simulink model "Substructuring"  (R2021a)
settings: Solver=ode8  StartTime=0.0  StopTime=31.2  FixedStep=dtfast  RelTol=1e-3
PreLoadFcn:
  | initializeSimulation;
InitFcn:
  | clear('all');
  | initializeSimulation;
undefined symbols (not defined in the file): adaptive, Ap, asiv, Bp, Cp, DiscIntNeverNeededParam, Dp, dtsim, f, ke, kgap, khard, learningrate, n1siv, n2siv, Ngap, nsiv, stiffdeg, strdegHmos, V1, w_80, x02, xgap, xy
libraries: raspberrypiNetworklib x2, instrumentlib x2, sldrtlib x1
settings Model: Creator=diego.mera  LastModifiedBy=diego.mera
settings SolverCC: PositivePriorityOrder=on
settings OptimizationCC: EnhancedBackFolding=on  PassReuseOutputArgsAs=Individual arguments  ZeroExternalMemoryAtStartup=off  ZeroInternalMemoryAtStartup=off  MaxStackSize=64  OptimizeBlockOrder=speed  DifferentSizesBufferReuse=on  OptimizationCustomize=off  EfficientTunableParamExpr=on
settings DebuggingCC: ParameterTunabilityLossMsg=error
settings HardwareCC: ProdBitPerPointer=32  ProdBitPerSizeT=32  ProdBitPerPtrDiffT=32  ProdLargestAtomicInteger=Long  ProdLargestAtomicFloat=Double  ProdWordSize=32  ProdLongLongMode=on  ProdHWDeviceType=ARM Compatible->ARM Cortex
settings RTWCC: SystemTargetFile=ert.tlc  HardwareBoard=Raspberry Pi  TLCOptions="-aInlineSetEventsForThisBaseRateFcn=TLC_FALSE -aSuppressMultiTaskScheduler=TLC_FALSE  -aRateBasedStepFcn=0"  TemplateMakefile=ert_default_tmf  Toolchain=GNU GCC Embedded Linux  BuildConfiguration=Faster Runs
settings CodeAppCC: ForceParamTrailComments=on  IgnoreCustomStorageClasses=off  OperatorAnnotations=on  SimulinkDataObjDesc=on  SFDataObjDesc=on  InsertBlockDesc=on
settings ERTTargetCC: SupportContinuousTime=on  SupportVariableSizeSignals=on  ExtModeTransport=2  ExtModeStaticAlloc=on  ExtModeMexFile=ext_xcp  ExtModeIntrfLevel=Level2 - Open

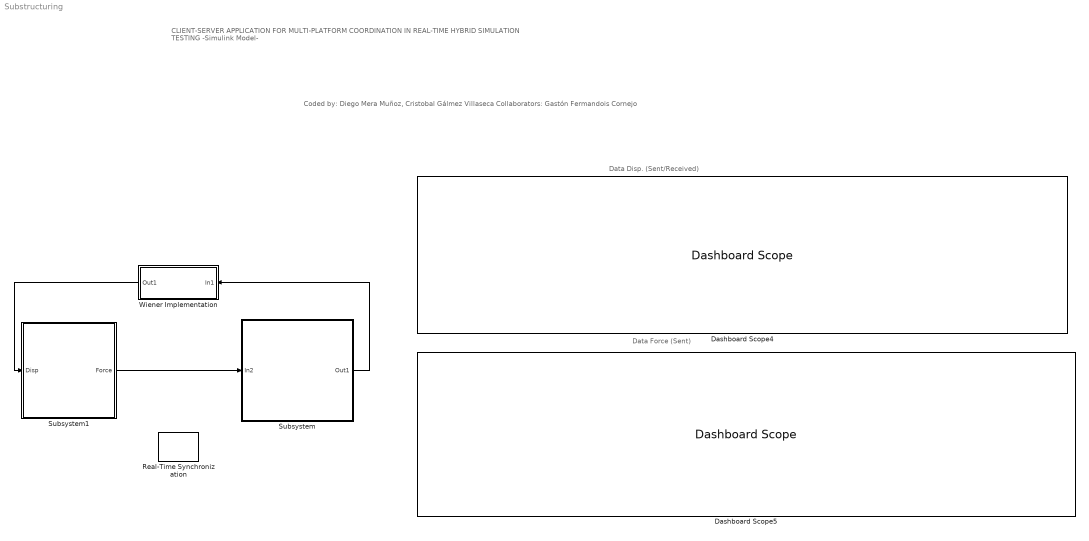
== system Substructuring ==
  note: Data Disp. (Sent/Received)
  note: Data Force (Sent)
  note: CLIENT-SERVER APPLICATION FOR MULTI-PLATFORM COORDINATION IN REAL-TIME HYBRID SIMULATION TESTING
      | -Simulink Model-
  note: Coded by: Diego Mera Muñoz, Cristobal Gálmez Villaseca
      | Collaborators: Gastón Fermandois Cornejo
  Dashboard Scope4 : DashboardScope  Ymin=-5  Ymax=5
  Dashboard Scope5 : DashboardScope  Ymin=-1.5e-5  Ymax=1e-5
  Real-Time Synchronization : sldrtlib/Real-Time Synchronization  SampleTime=dtsim  MaxMissedTicks=1000000  ShowMissedTicks=off  YieldWhenWaiting=off
  Subsystem : Subsystem
      mask Display: disp('NUMERICAL\nSUBSTRUCTURE')
  Subsystem1 : Subsystem
      mask Display: disp('EXPERIMENTAL\nSUBSTRUCTURE')
  Wiener Implementation : Subsystem
      mask Display: disp('DDMRT FILTER')
  wires:
  Subsystem1/1(Force) -> Subsystem/1(In2)
  Subsystem/1(Out1) -> Wiener Implementation/1(In1)
  Wiener Implementation/1(Out1) -> Subsystem1/1(Disp)

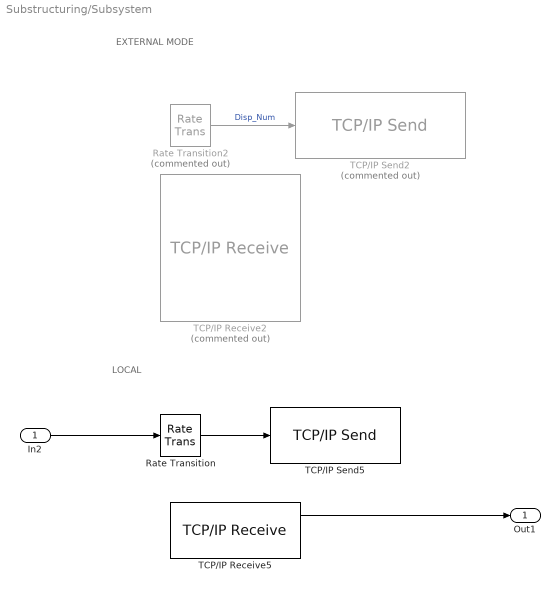
== system Substructuring/Subsystem ==
  note: EXTERNAL MODE
  note: LOCAL
  In2 : Inport
  Rate Transition : RateTransition  OutPortSampleTime=dtsim
  Rate Transition2 : RateTransition  Commented=on  OutPortSampleTime=dtsim
  TCP/IP Receive2 : raspberrypiNetworklib/TCP//IP Receive  Priority=2  Commented=on  Mode_=Client  LocalServerPort_=8090  RemoteAddr_=192.168.0.18  RemoteServerPort_=8090  DataType_=double  DataSize_=1  SampleTime_=dtsim  SimulateUsing=Code generation  ClientPortBindingSelection_=off  ClientPortToBind_=35000  BlockingMode_=on  BlockTimeout_=0.01  BlockPlatform=RASPBERRYPI
      settings: SourceProductBaseCode=RASPPI
  TCP/IP Receive5 : instrumentlib/TCP//IP Receive  Priority=1  Host=127.0.0.1  Port=8090  DataSize=1  EnableBlockingMode=off  Timeout=10  SampleTime=dtsim  DataType=double  ByteOrder=BigEndian  ASCIIFormatting=%f,  Terminator=LF
  TCP/IP Send2 : raspberrypiNetworklib/TCP//IP Send  Priority=1  Commented=on  Mode_=Client  LocalServerPort_=8090  RemoteAddr_=192.168.0.18  RemoteServerPort_=8090  SimulateUsing=Code generation  ClientPortBindingSelection_=off  ClientPortToBind_=35000  BlockingMode_=on  BlockTimeout_=0.02  BlockPlatform=RASPBERRYPI
      settings: SourceProductBaseCode=RASPPI
  TCP/IP Send5 : instrumentlib/TCP//IP Send  Priority=2  Host=127.0.0.1  Port=8090  EnableBlockingMode=off  Timeout=0.02  ByteOrder=BigEndian  TransferDelay=on
  Out1 : Outport
  wires:
  Rate Transition/1 -> TCP/IP Send5/1
  Rate Transition2/1 -> TCP/IP Send2/1  "Disp_Num"
  In2/1 -> Rate Transition/1
  TCP/IP Receive5/1 -> Out1/1

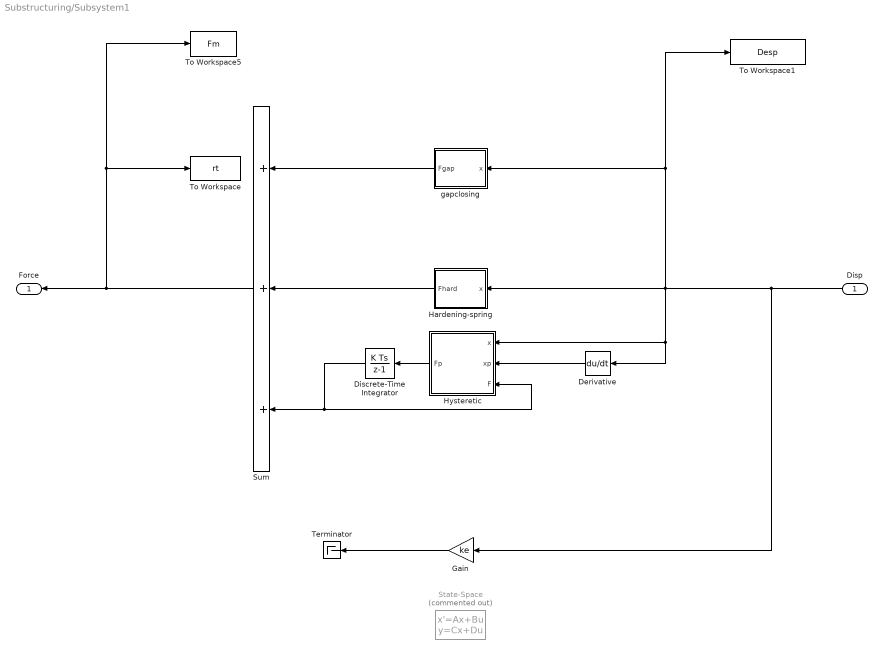
== system Substructuring/Subsystem1 ==
  Disp : Inport
  Derivative : Derivative
  Discrete-Time Integrator : DiscreteIntegrator  SampleTime=-1  ICPrevOutput=DiscIntNeverNeededParam  ICPrevScaledInput=DiscIntNeverNeededParam
  Gain : Gain  Gain=ke
  Hardening-spring : Subsystem
  Hysteretic : Subsystem
  State-Space : StateSpace  Commented=on  A=Ap  B=Bp  C=Cp  D=Dp  InitialCondition=0
  Sum : Sum  Inputs=+++
  Terminator : Terminator
  To Workspace : ToWorkspace  VariableName=rt  SaveFormat=Timeseries  SampleTime=-1
  To Workspace1 : ToWorkspace  VariableName=Desp  SaveFormat=Timeseries  SampleTime=-1
  To Workspace5 : ToWorkspace  VariableName=Fm  SaveFormat=Timeseries  SampleTime=-1
  gapclosing : Subsystem
  Force : Outport  VectorParamsAs1DForOutWhenUnconnected=off
  wires:
  gapclosing/1(Fgap) -> Sum/1
  Discrete-Time Integrator/1 -> Hysteretic/3(F), Sum/3
  Hardening-spring/1(Fhard) -> Sum/2
  Hysteretic/1(Fp) -> Discrete-Time Integrator/1
  Derivative/1 -> Hysteretic/2(xp)
  Disp/1 -> Gain/1, To Workspace1/1, gapclosing/1(x), Hysteretic/1(x), Derivative/1, Hardening-spring/1(x)
  Sum/1 -> To Workspace5/1, To Workspace/1, Force/1
  Gain/1 -> Terminator/1

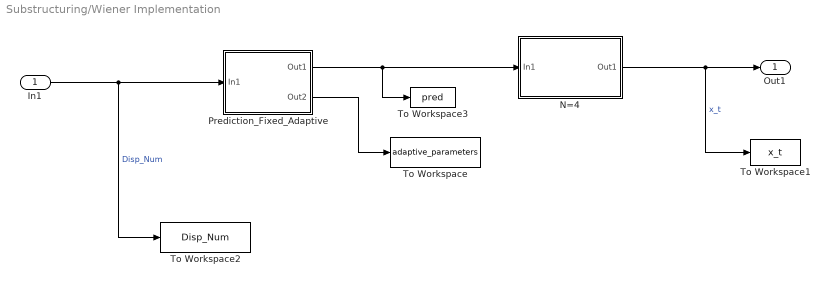
== system Substructuring/Wiener Implementation ==
  In1 : Inport
  N=4 : Subsystem
      mask Display: disp('MONOMIAL\nINTERPOLATION')
  Prediction_Fixed_Adaptive : Subsystem
      mask Display: disp('PREDICTION\n(Adaptive w)')
  To Workspace : ToWorkspace  VariableName=adaptive_parameters  SaveFormat=Timeseries  SampleTime=-1
  To Workspace1 : ToWorkspace  VariableName=x_t  SaveFormat=Timeseries  SampleTime=-1
  To Workspace2 : ToWorkspace  VariableName=Disp_Num  SaveFormat=Timeseries  SampleTime=-1
  To Workspace3 : ToWorkspace  VariableName=pred  SaveFormat=Timeseries  SampleTime=-1
  Out1 : Outport
  wires:
  In1/1 -> Prediction_Fixed_Adaptive/1(In1), To Workspace2/1  "Disp_Num"
  Prediction_Fixed_Adaptive/2(Out2) -> To Workspace/1
  N=4/1(Out1) -> To Workspace1/1, Out1/1  "x_t"
  Prediction_Fixed_Adaptive/1(Out1) -> To Workspace3/1, N=4/1(In1)

== system Substructuring/Subsystem1/Hardening-spring ==
  x : Inport
  Constant1 : Constant  Value=khard
  MATLAB Function : MATLAB Function  TreatAsAtomicUnit=on
  To Workspace : ToWorkspace  VariableName=Fhard  SaveFormat=Timeseries  SampleTime=-1
  Unit Delay : UnitDelay  SampleTime=-1  HasFrameUpgradeWarning=on
  Fhard : Outport  VectorParamsAs1DForOutWhenUnconnected=off
  wires:
  x/1 -> Unit Delay/1
  Constant1/1 -> MATLAB Function/2(khard)
  MATLAB Function/1(Fhard) -> Fhard/1, To Workspace/1
  Unit Delay/1 -> MATLAB Function/1(x)

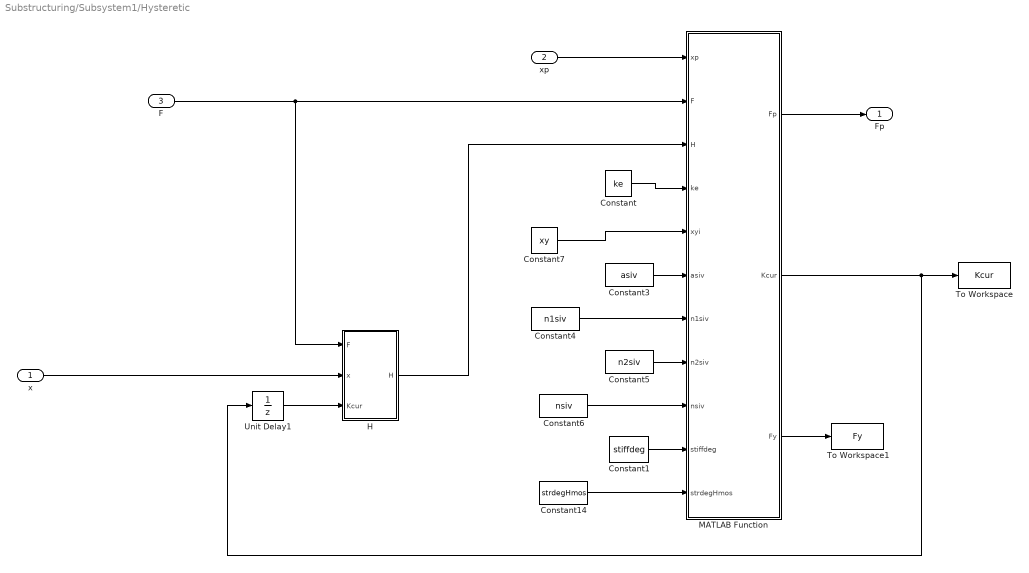
== system Substructuring/Subsystem1/Hysteretic ==
  x : Inport
  xp : Inport  Port=2
  F : Inport  Port=3
  Constant : Constant  Value=ke
  Constant1 : Constant  Value=stiffdeg
  Constant14 : Constant  Value=strdegHmos
  Constant3 : Constant  Value=asiv
  Constant4 : Constant  Value=n1siv
  Constant5 : Constant  Value=n2siv
  Constant6 : Constant  Value=nsiv
  Constant7 : Constant  Value=xy
  H : Subsystem
  MATLAB Function : MATLAB Function  TreatAsAtomicUnit=on
  To Workspace : ToWorkspace  VariableName=Kcur  SaveFormat=Timeseries  SampleTime=-1
  To Workspace1 : ToWorkspace  VariableName=Fy  SaveFormat=Timeseries  SampleTime=-1
  Unit Delay1 : UnitDelay  InitialCondition=ke  SampleTime=-1  HasFrameUpgradeWarning=on
  Fp : Outport  VectorParamsAs1DForOutWhenUnconnected=off
  wires:
  MATLAB Function/1(Fp) -> Fp/1
  MATLAB Function/2(Kcur) -> To Workspace/1, Unit Delay1/1
  x/1 -> H/2(x)
  xp/1 -> MATLAB Function/1(xp)
  Constant/1 -> MATLAB Function/4(ke)
  Constant7/1 -> MATLAB Function/5(xyi)
  Constant1/1 -> MATLAB Function/10(stiffdeg)
  Constant3/1 -> MATLAB Function/6(asiv)
  Constant4/1 -> MATLAB Function/7(n1siv)
  Constant5/1 -> MATLAB Function/8(n2siv)
  Constant6/1 -> MATLAB Function/9(nsiv)
  H/1(H) -> MATLAB Function/3(H)
  Unit Delay1/1 -> H/3("Kcur ")
  F/1 -> MATLAB Function/2(F), H/1(F)
  MATLAB Function/3(Fy) -> To Workspace1/1
  Constant14/1 -> MATLAB Function/11(strdegHmos)

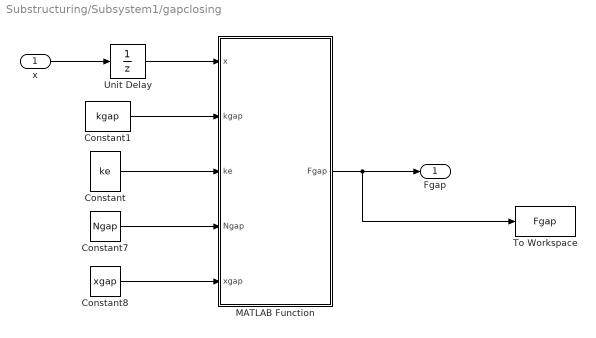
== system Substructuring/Subsystem1/gapclosing ==
  x : Inport
  Constant : Constant  Value=ke
  Constant1 : Constant  Value=kgap
  Constant7 : Constant  Value=Ngap
  Constant8 : Constant  Value=xgap
  MATLAB Function : MATLAB Function  TreatAsAtomicUnit=on
  To Workspace : ToWorkspace  VariableName=Fgap  SaveFormat=Timeseries  SampleTime=-1
  Unit Delay : UnitDelay  SampleTime=-1  HasFrameUpgradeWarning=on
  Fgap : Outport  VectorParamsAs1DForOutWhenUnconnected=off
  wires:
  Constant7/1 -> MATLAB Function/4(Ngap)
  MATLAB Function/1(Fgap) -> To Workspace/1, Fgap/1
  Constant1/1 -> MATLAB Function/2(kgap)
  Constant8/1 -> MATLAB Function/5(xgap)
  Constant/1 -> MATLAB Function/3(ke)
  x/1 -> Unit Delay/1
  Unit Delay/1 -> MATLAB Function/1(x)

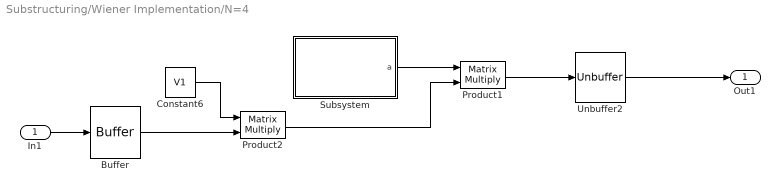
== system Substructuring/Wiener Implementation/N=4 ==
  In1 : Inport
  Buffer : Buffer  N=4  V=3  OutputFrames=off
  Constant6 : Constant  Value=V1
  Product1 : Product  Multiplication=Matrix(*)
  Product2 : Product  Multiplication=Matrix(*)
  Subsystem : Subsystem
  Unbuffer2 : Unbuffer
  Out1 : Outport
  wires:
  Product2/1 -> Product1/2
  Constant6/1 -> Product2/1
  Unbuffer2/1 -> Out1/1
  In1/1 -> Buffer/1
  Product1/1 -> Unbuffer2/1
  Subsystem/1(a) -> Product1/1
  Buffer/1 -> Product2/2

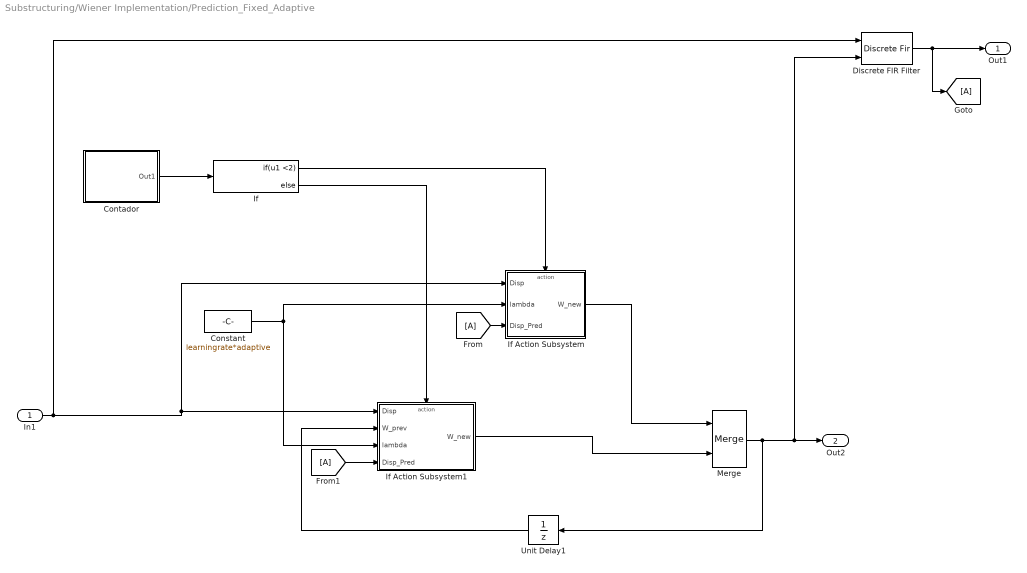
== system Substructuring/Wiener Implementation/Prediction_Fixed_Adaptive ==
  In1 : Inport
  Constant : Constant  Value=learningrate*adaptive
  Contador : Subsystem
      mask Display: disp('Contador')
  Discrete FIR Filter : DiscreteFir  CoefSource=Input port  SampleTime=dtsim
      settings: InputPortMap=u0,u1
  If : If  IfExpression=u1 <2
  If Action Subsystem : Subsystem  TreatAsAtomicUnit=on
  If Action Subsystem1 : Subsystem  TreatAsAtomicUnit=on
  Merge : Merge
  Unit Delay1 : UnitDelay  SampleTime=-1  HasFrameUpgradeWarning=on
  Out1 : Outport
  Out2 : Outport  Port=2
  wires:
  If Action Subsystem/1(W_new) -> Merge/1
  In1/1 -> Discrete FIR Filter/1, If Action Subsystem/1(Disp), If Action Subsystem1/1(Disp)
  If Action Subsystem1/1(W_new) -> Merge/2
  If/1 -> If Action Subsystem/Action
  Unit Delay1/1 -> If Action Subsystem1/2(W_prev)
  Merge/1 -> Discrete FIR Filter/2, Out2/1, Unit Delay1/1
  If/2 -> If Action Subsystem1/Action
  Contador/1(Out1) -> If/1
  Constant/1 -> If Action Subsystem1/3(lambda), If Action Subsystem/2(lambda)
  Discrete FIR Filter/1 -> [A], Out1/1
  [A] -> If Action Subsystem/3(Disp_Pred)
  [A] -> If Action Subsystem1/4(Disp_Pred)

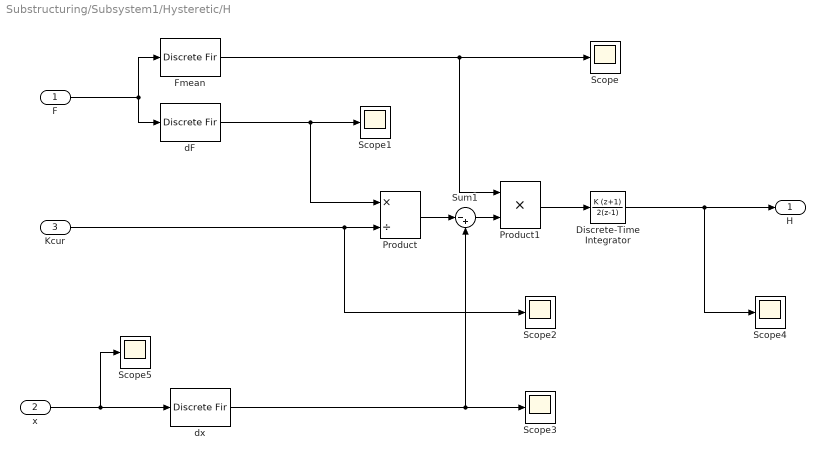
== system Substructuring/Subsystem1/Hysteretic/H ==
  F : Inport
  x : Inport  Port=2
  "Kcur " : Inport  Port=3
  Discrete-Time Integrator : DiscreteIntegrator  IntegratorMethod=Accumulation: Trapezoidal  SampleTime=-1  ICPrevOutput=DiscIntNeverNeededParam  ICPrevScaledInput=DiscIntNeverNeededParam
  Fmean : DiscreteFir
  Product : Product  Inputs=*/
  Product1 : Product
  Scope{,1..5} (6 alike) : Scope
  Sum1 : Sum  Inputs=|-+
  dF : DiscreteFir  Coefficients=[1 -1]
  dx : DiscreteFir  Coefficients=[1 -1]
  H : Outport  VectorParamsAs1DForOutWhenUnconnected=off
  wires:
  dF/1 -> Scope1/1, Product/1
  "Kcur "/1 -> Scope2/1, Product/2
  Product1/1 -> Discrete-Time Integrator/1
  Sum1/1 -> Product1/2
  x/1 -> Scope5/1, dx/1
  F/1 -> Fmean/1, dF/1
  Discrete-Time Integrator/1 -> Scope4/1, H/1
  Product/1 -> Sum1/1
  dx/1 -> Scope3/1, Sum1/2
  Fmean/1 -> Scope/1, Product1/1

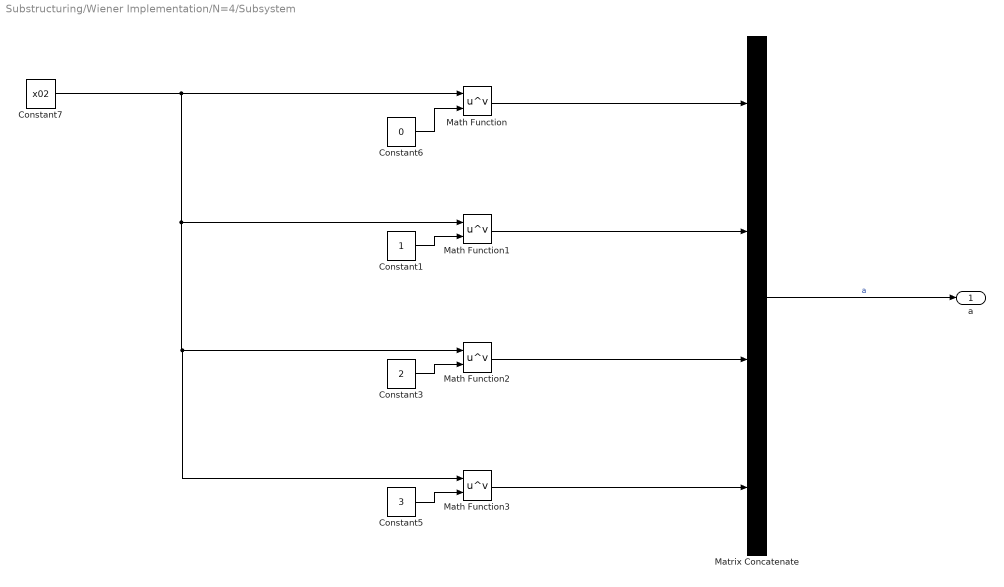
== system Substructuring/Wiener Implementation/N=4/Subsystem ==
  Constant1 : Constant
  Constant3 : Constant  Value=2
  Constant5 : Constant  Value=3
  Constant6 : Constant  Value=0
  Constant7 : Constant  Value=x02
  Math Function{,1..3} (4 alike) : Math  Operator=pow  SaturateOnIntegerOverflow=on
  Matrix Concatenate : Concatenate  NumInputs=4  Mode=Multidimensional array  ConcatenateDimension=2
  a : Outport
  wires:
  Constant6/1 -> Math Function/2
  Constant1/1 -> Math Function1/2
  Constant3/1 -> Math Function2/2
  Constant5/1 -> Math Function3/2
  Math Function/1 -> Matrix Concatenate/1
  Math Function1/1 -> Matrix Concatenate/2
  Math Function2/1 -> Matrix Concatenate/3
  Math Function3/1 -> Matrix Concatenate/4
  Matrix Concatenate/1 -> a/1  "a"
  Constant7/1 -> Math Function3/1, Math Function2/1, Math Function1/1, Math Function/1

== system Substructuring/Wiener Implementation/Prediction_Fixed_Adaptive/Contador ==
  Add : Sum
  Constant1 : Constant
  Unit Delay : UnitDelay  SampleTime=-1  HasFrameUpgradeWarning=on
  Out1 : Outport
  wires:
  Unit Delay/1 -> Add/2
  Constant1/1 -> Add/1
  Add/1 -> Out1/1, Unit Delay/1

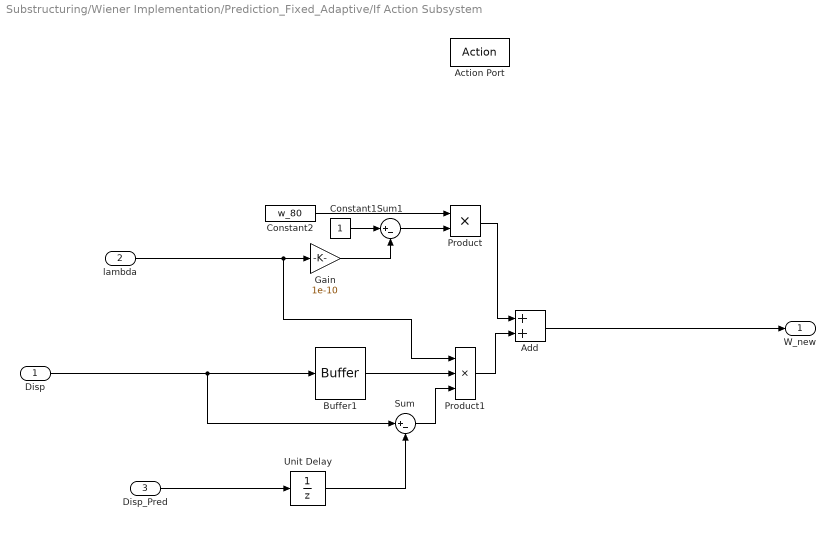
== system Substructuring/Wiener Implementation/Prediction_Fixed_Adaptive/If Action Subsystem ==
  Disp : Inport
  lambda : Inport  Port=2
  Disp_Pred : Inport  Port=3
  Action Port : ActionPort  ActionPortLabel=if(u1 <2)
  Add : Sum
  Buffer1 : Buffer  N=8  V=7  OutputFrames=off
  Constant1 : Constant
  Constant2 : Constant  Value=w_80
  Gain : Gain  Gain=1e-10
  Product : Product
  Product1 : Product  Inputs=3
  Sum : Sum  Inputs=|+-
  Sum1 : Sum  Inputs=|+-
  Unit Delay : UnitDelay  SampleTime=-1  HasFrameUpgradeWarning=on
  W_new : Outport
  wires:
  lambda/1 -> Product1/1, Gain/1
  Gain/1 -> Sum1/2
  Add/1 -> W_new/1
  Constant2/1 -> Product/1
  Buffer1/1 -> Product1/2
  Product1/1 -> Add/2
  Product/1 -> Add/1
  Disp/1 -> Buffer1/1, Sum/1
  Sum1/1 -> Product/2
  Sum/1 -> Product1/3
  Unit Delay/1 -> Sum/2
  Constant1/1 -> Sum1/1
  Disp_Pred/1 -> Unit Delay/1

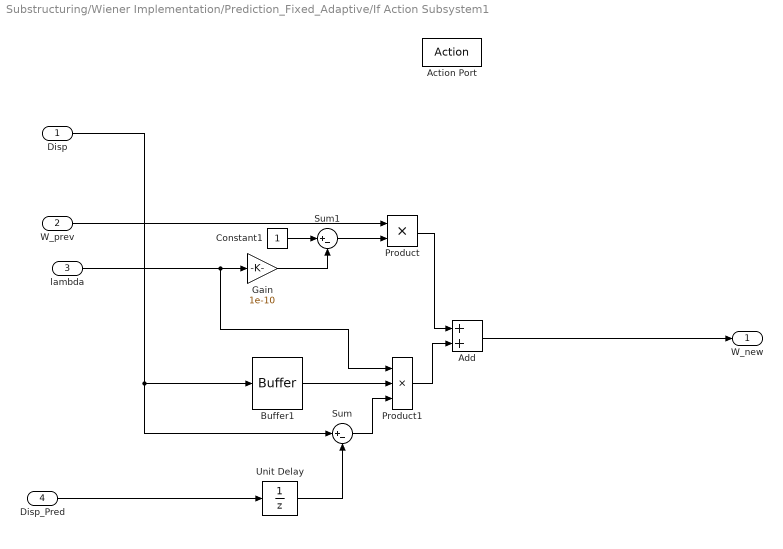
== system Substructuring/Wiener Implementation/Prediction_Fixed_Adaptive/If Action Subsystem1 ==
  Disp : Inport
  W_prev : Inport  Port=2
  lambda : Inport  Port=3
  Disp_Pred : Inport  Port=4
  Action Port : ActionPort  ActionPortLabel=else
  Add : Sum
  Buffer1 : Buffer  N=8  V=7  OutputFrames=off
  Constant1 : Constant
  Gain : Gain  Gain=1e-10
  Product : Product
  Product1 : Product  Inputs=3
  Sum : Sum  Inputs=|+-
  Sum1 : Sum  Inputs=|+-
  Unit Delay : UnitDelay  SampleTime=-1  HasFrameUpgradeWarning=on
  W_new : Outport
  wires:
  lambda/1 -> Product1/1, Gain/1
  Gain/1 -> Sum1/2
  Add/1 -> W_new/1
  W_prev/1 -> Product/1
  Buffer1/1 -> Product1/2
  Product1/1 -> Add/2
  Product/1 -> Add/1
  Disp/1 -> Buffer1/1, Sum/1
  Sum1/1 -> Product/2
  Sum/1 -> Product1/3
  Unit Delay/1 -> Sum/2
  Constant1/1 -> Sum1/1
  Disp_Pred/1 -> Unit Delay/1

== matlab function Substructuring/Subsystem1/Hardening-spring/MATLAB Function ==
  data: x input; Fhard output; khard input
function Fhard  = hardening(x,khard)
Fhard=khard*(x^3);

== matlab function Substructuring/Subsystem1/Hysteretic/MATLAB Function ==
  data: xp input; F input; H input; Fp output; ke input; xyi input; asiv input; n1siv input; n2siv input; nsiv input; stiffdeg input; Kcur output; Fy output; strdegHmos input
function [Fp,Kcur,Fy] = stiffdegradation(xp,F,H,ke,xyi,asiv,n1siv,n2siv,nsiv,stiffdeg,strdegHmos)

Kcur=((exp(-stiffdeg*H))-asiv)*ke; 
Fyi=(1-asiv)*ke*xyi;
Fy=Fyi*(1+strdegHmos*H)^-1;
if Fy<=0.01*Fyi
    Fy=Fyi*0.01;
end
Khyst=Kcur*(1-abs(F/Fy)^(nsiv)*(n1siv*sign(F*xp)+n2siv));
Fp=Khyst*xp;

== matlab function Substructuring/Subsystem1/gapclosing/MATLAB Function ==
  data: x input; Fgap output; kgap input; ke input; Ngap input; xgap input
function Fgap  = gapclosing(x,kgap,ke,Ngap,xgap)
if abs(x)<=xgap
    Fgap=0;
else
    Fgap=kgap*ke*Ngap*(abs(x)-xgap)^(Ngap-1)*x;
end
